simulink model "zbiorniki"  (R2015b)
settings: Solver=ode4  StartTime=0.0  StopTime=200.0  FixedStep=0.05  RelTol=1e-3
InitFcn:
  | run init.m
values from neighbouring files (symbols this model uses):
  H2 = 40    [init.m]
  HH2 = 50    [init.m]
  L2 = 10    [init.m]
  LL2 = 5    [init.m]
  r = 1    [init.m]
libraries: simulink x4
settings Model: Creator=Piotrek  LastModifiedBy=Piotrek

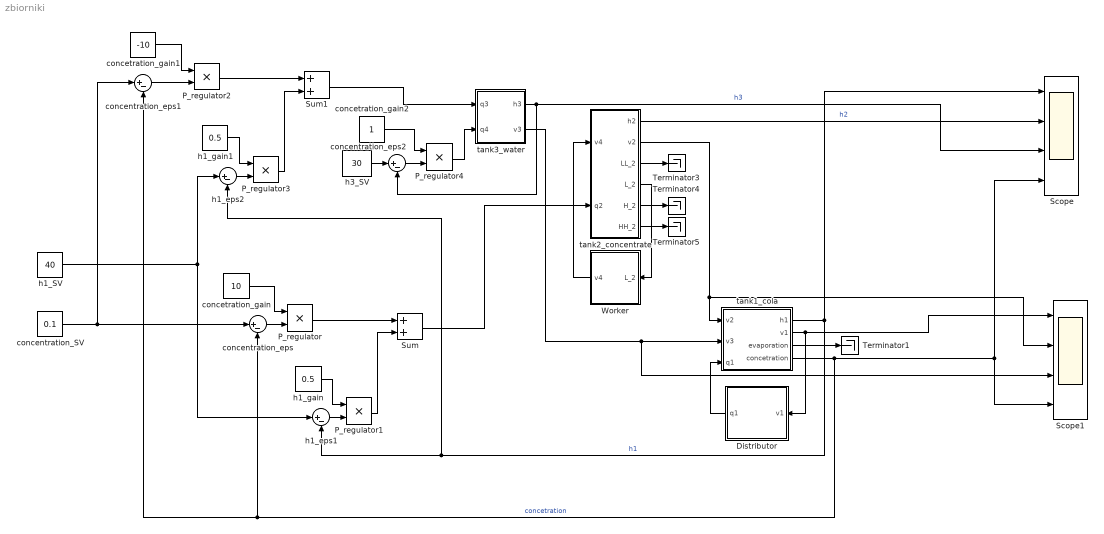
== system zbiorniki ==
  Distributor : Subsystem
  P_regulator{,1..4} (5 alike) : Product  Inputs=**
  Scope : Scope  NumInputPorts=4
  Scope1 : Scope  NumInputPorts=4
  Sum : Sum
  Sum1 : Sum
  Terminator{1,3..5} (4 alike) : Terminator
  Worker : Subsystem
  concentration_SV : Constant  Value=0.1
  concentration_eps : Sum  Inputs=|+-
  concentration_eps1 : Sum  Inputs=|+-
  concentration_eps2 : Sum  Inputs=|+-
  concetration_gain : Constant  Value=10
  concetration_gain1 : Constant  Value=-10
  concetration_gain2 : Constant
  h1_SV : Constant  Value=40
  h1_eps1 : Sum  Inputs=|+-
  h1_eps2 : Sum  Inputs=|+-
  h1_gain : Constant  Value=0.5
  h1_gain1 : Constant  Value=0.5
  h3_SV : Constant  Value=30
  tank1_cola : Subsystem
  tank2_concentrate : Subsystem
  tank3_water : Subsystem
  wires:
  tank2_concentrate/2(v2) -> tank1_cola/1(v2), Scope1/2
  tank3_water/2(v3) -> Scope1/3, tank1_cola/2(v3)
  tank1_cola/2(v1) -> Scope1/1, Distributor/1(v1)
  tank3_water/1(h3) -> Scope/3, concentration_eps2/2  "h3"
  tank2_concentrate/1(h2) -> Scope/2  "h2"
  tank1_cola/1(h1) -> Scope/1, h1_eps1/2, h1_eps2/2  "h1"
  tank1_cola/4(concetration) -> concentration_eps/2, concentration_eps1/2, Scope/4, Scope1/4  "concetration"
  Distributor/1(q1) -> tank1_cola/3(q1)
  tank2_concentrate/3(LL_2) -> Terminator3/1
  tank2_concentrate/5(H_2) -> Terminator4/1
  tank2_concentrate/6(HH_2) -> Terminator5/1
  tank2_concentrate/4(L_2) -> Worker/1(L_2)
  Worker/1(v4) -> tank2_concentrate/1(v4)
  Sum1/1 -> tank3_water/1(q3)
  concetration_gain/1 -> P_regulator/1
  concentration_eps/1 -> P_regulator/2
  P_regulator/1 -> Sum/1
  Sum/1 -> tank2_concentrate/2(q2)
  h1_SV/1 -> h1_eps1/1, h1_eps2/1
  tank1_cola/3(evaporation) -> Terminator1/1
  h1_gain/1 -> P_regulator1/1
  h1_eps1/1 -> P_regulator1/2
  P_regulator1/1 -> Sum/2
  concentration_SV/1 -> concentration_eps1/1, concentration_eps/1
  concetration_gain1/1 -> P_regulator2/1
  concentration_eps1/1 -> P_regulator2/2
  P_regulator2/1 -> Sum1/1
  h1_gain1/1 -> P_regulator3/1
  h1_eps2/1 -> P_regulator3/2
  P_regulator3/1 -> Sum1/2
  concetration_gain2/1 -> P_regulator4/1
  concentration_eps2/1 -> P_regulator4/2
  h3_SV/1 -> concentration_eps2/1
  P_regulator4/1 -> tank3_water/2(q4)

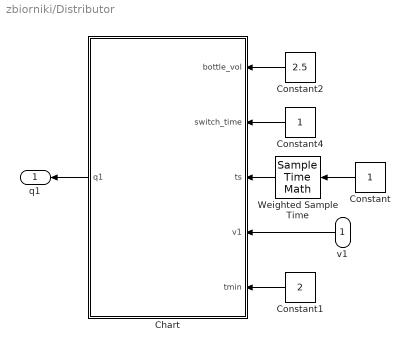
== system zbiorniki/Distributor ==
  v1 : Inport
  Chart : Stateflow chart  TreatAsAtomicUnit=on
  Constant : Constant
  Constant1 : Constant  Value=2
  Constant2 : Constant  Value=2.5
  Constant4 : Constant
  Weighted Sample Time : SampleTimeMath  TsampMathOp=Ts Only  weightValue=1
  q1 : Outport
  wires:
  Constant/1 -> Weighted Sample Time/1
  Weighted Sample Time/1 -> Chart/3(ts)
  v1/1 -> Chart/4(v1)
  Constant1/1 -> Chart/5(tmin)
  Constant2/1 -> Chart/1(bottle_vol)
  Constant4/1 -> Chart/2(switch_time)
  Chart/1(q1) -> q1/1

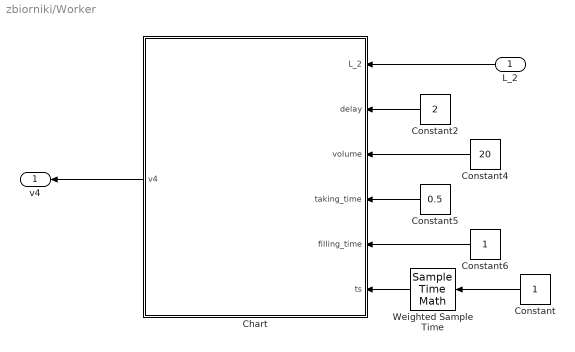
== system zbiorniki/Worker ==
  L_2 : Inport
  Chart : Stateflow chart  TreatAsAtomicUnit=on
  Constant : Constant
  Constant2 : Constant  Value=2
  Constant4 : Constant  Value=20
  Constant5 : Constant  Value=0.5
  Constant6 : Constant
  Weighted Sample Time : SampleTimeMath  TsampMathOp=Ts Only  weightValue=1
  v4 : Outport
  wires:
  Constant5/1 -> Chart/4(taking_time)
  Constant6/1 -> Chart/5(filling_time)
  Constant/1 -> Weighted Sample Time/1
  Constant4/1 -> Chart/3(volume)
  Constant2/1 -> Chart/2(delay)
  L_2/1 -> Chart/1(L_2)
  Weighted Sample Time/1 -> Chart/6(ts)
  Chart/1(v4) -> v4/1

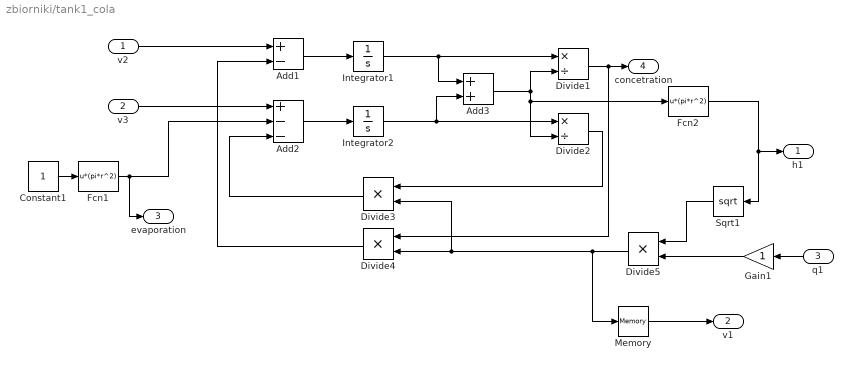
== system zbiorniki/tank1_cola ==
  v2 : Inport
  v3 : Inport  Port=2
  q1 : Inport  Port=3
  Add1 : Sum  Inputs=+-
  Add2 : Sum  Inputs=+--
  Add3 : Sum
  Constant1 : Constant
  Divide1 : Product  Inputs=*/
  Divide2 : Product  Inputs=*/
  Divide3 : Product
  Divide4 : Product
  Divide5 : Product
  Fcn1 : Fcn  Expr=u*(pi*r^2)
  Fcn2 : Fcn  Expr=u*(pi*r^2)
  Gain1 : Gain
  Integrator1 : Integrator  InitialCondition=5/(pi*r^2)  LimitOutput=on  LowerSaturationLimit=0
  Integrator2 : Integrator  InitialCondition=10/(pi*r^2)  LimitOutput=on  LowerSaturationLimit=0
  Memory : Memory
  Sqrt1 : Sqrt  SaturateOnIntegerOverflow=on
  h1 : Outport
  v1 : Outport  Port=2
  evaporation : Outport  Port=3
  concetration : Outport  Port=4
  wires:
  v2/1 -> Add1/1
  v3/1 -> Add2/1
  Fcn1/1 -> Add2/2, evaporation/1
  Constant1/1 -> Fcn1/1
  Add1/1 -> Integrator1/1
  Add2/1 -> Integrator2/1
  Integrator1/1 -> Divide1/1, Add3/1
  Integrator2/1 -> Divide2/1, Add3/2
  Add3/1 -> Fcn2/1, Divide2/2, Divide1/2
  q1/1 -> Gain1/1
  Divide3/1 -> Add2/3
  Divide4/1 -> Add1/2
  Sqrt1/1 -> Divide5/1
  Gain1/1 -> Divide5/2
  Fcn2/1 -> h1/1, Sqrt1/1
  Divide5/1 -> Memory/1, Divide3/2, Divide4/2
  Divide2/1 -> Divide3/1
  Divide1/1 -> Divide4/1, concetration/1
  Memory/1 -> v1/1

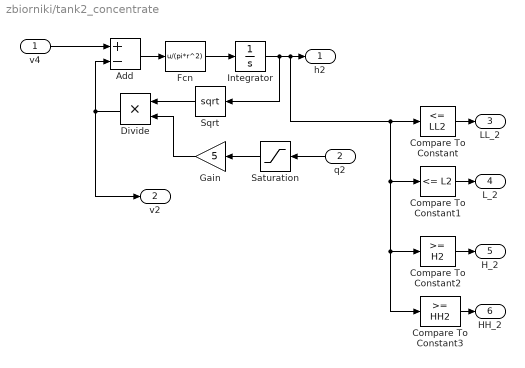
== system zbiorniki/tank2_concentrate ==
  v4 : Inport
  q2 : Inport  Port=2
  Add : Sum  Inputs=+-
  Compare To Constant : simulink/Logic and Bit Operations/Compare To Constant  relop=<=  const=LL2  OutDataTypeStr=boolean
  Compare To Constant1 : simulink/Logic and Bit Operations/Compare To Constant  relop=<=  const=L2  OutDataTypeStr=boolean
  Compare To Constant2 : simulink/Logic and Bit Operations/Compare To Constant  relop=>=  const=H2  OutDataTypeStr=boolean
  Compare To Constant3 : simulink/Logic and Bit Operations/Compare To Constant  relop=>=  const=HH2  OutDataTypeStr=boolean
  Divide : Product
  Fcn : Fcn  Expr=u/(pi*r^2)
  Gain : Gain  Gain=5
  Integrator : Integrator  InitialCondition=20  LimitOutput=on  LowerSaturationLimit=0
  Saturation : Saturate  UpperLimit=1  LowerLimit=0
  Sqrt : Sqrt  SaturateOnIntegerOverflow=on
  h2 : Outport
  v2 : Outport  Port=2
  LL_2 : Outport  Port=3
  L_2 : Outport  Port=4
  H_2 : Outport  Port=5
  HH_2 : Outport  Port=6
  wires:
  Integrator/1 -> Compare To Constant1/1, Compare To Constant2/1, Compare To Constant3/1, Compare To Constant/1, h2/1, Sqrt/1
  q2/1 -> Saturation/1
  Add/1 -> Fcn/1
  Fcn/1 -> Integrator/1
  v4/1 -> Add/1
  Divide/1 -> v2/1, Add/2
  Sqrt/1 -> Divide/1
  Compare To Constant/1 -> LL_2/1
  Compare To Constant1/1 -> L_2/1
  Compare To Constant2/1 -> H_2/1
  Compare To Constant3/1 -> HH_2/1
  Saturation/1 -> Gain/1
  Gain/1 -> Divide/2

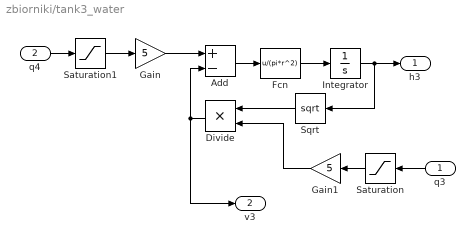
== system zbiorniki/tank3_water ==
  q3 : Inport
  q4 : Inport  Port=2
  Add : Sum  Inputs=+-
  Divide : Product
  Fcn : Fcn  Expr=u/(pi*r^2)
  Gain : Gain  Gain=5
  Gain1 : Gain  Gain=5
  Integrator : Integrator  InitialCondition=10
  Saturation : Saturate  UpperLimit=1  LowerLimit=0
  Saturation1 : Saturate  UpperLimit=1  LowerLimit=0
  Sqrt : Sqrt  SaturateOnIntegerOverflow=on
  h3 : Outport
  v3 : Outport  Port=2
  wires:
  Fcn/1 -> Integrator/1
  Add/1 -> Fcn/1
  q3/1 -> Saturation/1
  Integrator/1 -> Sqrt/1, h3/1
  Gain/1 -> Add/1
  Divide/1 -> Add/2, v3/1
  Sqrt/1 -> Divide/1
  q4/1 -> Saturation1/1
  Saturation/1 -> Gain1/1
  Gain1/1 -> Divide/2
  Saturation1/1 -> Gain/1

== stateflow chart zbiorniki/Distributor/Chart ==
  state Start
  state Filling_bottle
    en: t=0;
    q1=1;
    vol=0;
    du: vol=vol+v1*ts;
    t=t+ts;
    ex: q1=0;
  state Waiting_for_new_bottle
    en:t2=0;
    du: t=t+ts;
    t2=t+ts;
  (default) -> Start
  Start -> Filling_bottle
  Waiting_for_new_bottle -> Filling_bottle : [t>=tmin&t2>=switch_time]
  Filling_bottle -> Waiting_for_new_bottle : [vol>=bottle_vol]
  data: bottle_vol input; switch_time input; ts input; v1 input; tmin input; q1 output; t2 local; t local; vol local

== stateflow chart zbiorniki/Worker/Chart ==
  state Stand_by
  state Waiting_for_worker
    entry: t = delay;
    during: t = t - ts;
  state Taking_bottle
    entry: t1 = taking_time;
    during: t1 = t - ts;
  state Filling_tank
    entry: v4=volume/filling_time;
    t2=filling_time;
    du: t2 = t2 - ts;
    exit: v4=0
  (default) -> Stand_by
  Filling_tank -> Stand_by [order 2] : [t2<=0&L_2==0]
  Stand_by -> Waiting_for_worker : [L_2==1]
  Waiting_for_worker -> Taking_bottle : [t<=0]
  Filling_tank -> Taking_bottle [order 1] : [t2<=0&L_2==1]
  Taking_bottle -> Filling_tank : [t1<=0]
  data: L_2 input; delay input; volume input; taking_time input; filling_time input; ts input; t1 local; t local; t2 local; v4 output
